simulink model "spareparts"  (R2021b)
settings: Solver=VariableStepAuto  StartTime=0.0  StopTime=10.0  RelTol=1e-3
undefined symbols (not defined in the file or in its folder): wt
settings Model: Creator=tedbrekken  LastModifiedBy=tedbrekken

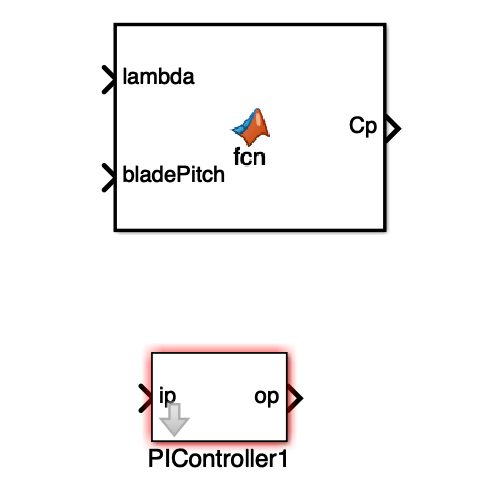
[thumbnail: Simulink's stored preview of the top-level diagram]
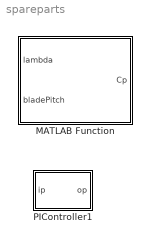
== system spareparts ==
  MATLAB Function : MATLAB Function  TreatAsAtomicUnit=on
  PIController1 : Subsystem  mask{kp=wt.speedcontroller.kp, ki=wt.speedcontroller.ki, kt=wt.speedcontroller.kt, upperLimit=wt.speedcontroller.upperLimit, lowerLimit=wt.speedcontroller.lowerLimit, int_0=wt.speedcontroller.int_0}
      mask prompts: kp "Proportional gain"; ki "Integral gain"; kt "Windup gain"; upperLimit "Upper limit"; lowerLimit "Lower limit"; int_0 "Initial condition"

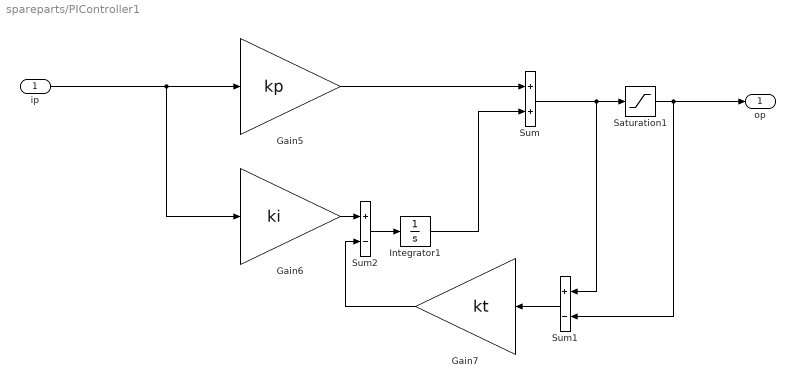
== system spareparts/PIController1 ==
  ip : Inport
  Gain5 : Gain  Gain=kp
  Gain6 : Gain  Gain=ki
  Gain7 : Gain  Gain=kt
  Integrator1 : Integrator  InitialCondition=int_0
  Saturation1 : Saturate  UpperLimit=upperLimit  LowerLimit=lowerLimit
  Sum : Sum
  Sum1 : Sum  Inputs=+-
  Sum2 : Sum  Inputs=+-
  op : Outport
  wires:
  Sum2/1 -> Integrator1/1
  Integrator1/1 -> Sum/2
  Gain7/1 -> Sum2/2
  Sum1/1 -> Gain7/1
  Gain6/1 -> Sum2/1
  ip/1 -> Gain6/1, Gain5/1
  Saturation1/1 -> op/1, Sum1/2
  Gain5/1 -> Sum/1
  Sum/1 -> Sum1/1, Saturation1/1

== matlab function spareparts/MATLAB Function ==
  data: lambda input; Cp output; bladePitch input
function Cp = fcn(lambda,bladePitch)

% https://www.mathworks.com/help/physmod/sps/powersys/ref/windturbine.html

c = [...
    0.5176 ...
    116 ...
    0.4 ...
    5 ...
    21 ...
    0.0068];

lambdaai = 1/( 1/(lambda+0.08*bladePitch) - 0.035/(bladePitch^3+1) );

Cp = c(1)*(c(2)/lambdaai-c(3)*bladePitch-c(4))*exp(-c(5)/lambdaai) + c(6)*lambda;
